simulink model "interpolation_nD_TestGen38"  (R2017b)
settings: Solver=FixedStepDiscrete  StartTime=0.0  StopTime=10.0  RelTol=1e-3
settings Model: Creator=ktrinh  LastModifiedBy=ktrinh
settings DebuggingCC: ParameterOverflowMsg=none

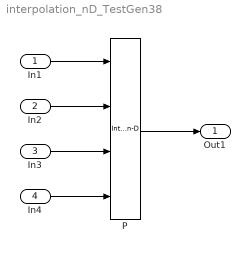
== system interpolation_nD_TestGen38 ==
  In1 : Inport  OutMin=0  OutMax=2  OutDataTypeStr=Bus: kfBus  PortDimensions=1  BusOutputAsStruct=on
  In2 : Inport  Port=2  OutMin=0  OutMax=5  OutDataTypeStr=Bus: kfBus  BusOutputAsStruct=on
  In3 : Inport  Port=3  OutMin=0  OutMax=3
  In4 : Inport  Port=4  PortDimensions=[2 5 3]
  P : Interpolation_n-D  InitFcn=|  NumberOfTableDimensions=3  TableSource=Input port  InterpMethod=Flat  ExtrapMethod=Clip  RequireIndexFractionAsBus=on  NumSelectionDims=1  OutDataTypeStr=int32  InternalRulePriority=Speed  RndMeth=Nearest
      | elems(1) = Simulink.BusElement;
      | elems(1).Name = 'Index';
      | elems(1).DataType = 'int8';
      | elems(2) = Simulink.BusElement;
      | elems(2).Name = 'Fraction';
      | elems(2).DataType = 'double';
      | kfBus = Simulink.Bus;
      | kfBus.Elements = elems;
      | clear elems;
      | assignin('base', 'kfBus', kfBus);
      settings: InputPortMap=u0,u1,u2,p2
  Out1 : Outport
  wires:
  In1/1 -> P/1
  In2/1 -> P/2
  In3/1 -> P/3
  In4/1 -> P/4
  P/1 -> Out1/1
